simulink model "DIPCRT"  (R2015a)
settings: Solver=ode23  SolverMode=SingleTasking  StartTime=0.0  StopTime=3  FixedStep=1e-3  RelTol=1e-3
values from neighbouring files (symbols this model uses):
  deltas = 1000    [DIPCRTinit.m]
  deltav = 5000    [DIPCRTinit.m]
  ds = 1000    [DIPCRTinit.m]
  dv = 5000    [DIPCRTinit.m]
  g = [0;0;0]    [DIPCRTinit.m]
  j0 = 1    [DIPCRTinit.m]
  j1 = 10    [DIPCRTinit.m]
  j2 = 10    [DIPCRTinit.m]
  j3 = 10    [DIPCRTinit.m]
  j4 = 10    [DIPCRTinit.m]
  jv = 1    [DIPCRTinit.m]
  kappas = 2000    [DIPCRTinit.m]
  kappav = 20000    [DIPCRTinit.m]
  kpr = 500    [DIPCRTinit.m]
  kpt = 500    [DIPCRTinit.m]
  ks = 2000    [DIPCRTinit.m]
  kv = 30    [DIPCRTinit.m]
  m0 = 10    [DIPCRTinit.m]
  m1 = 10    [DIPCRTinit.m]
  m2 = 10    [DIPCRTinit.m]
  m3 = 10    [DIPCRTinit.m]
  m4 = 10    [DIPCRTinit.m]
  mv = 10    [DIPCRTinit.m]
libraries: aerolibutil x22, dspinverses x3, aerolibtransform2 x2, simulink x2
(part 2 of 2)

== matlab function DIPCRT/Interaction dynamics1/MATLAB Function ==
  data: r parameter; A output; x input
function A = ConstraintMatrix(r,x)
A = [-eye(3) skew_sm(quatrot(x(4:7),r(1:3))) eye(3) zeros(3,21);
        zeros(3) -eye(3) zeros(3) eye(3) zeros(3,18);
        -eye(3) skew_sm(quatrot(x(4:7),r(4:6))) zeros(3,6) eye(3) zeros(3,15);
        zeros(3) -eye(3) zeros(3,9) eye(3) zeros(3,12);
        -eye(3) skew_sm(quatrot(x(4:7),r(7:9))) zeros(3,12) eye(3) zeros(3,9);
        zeros(3) -eye(3) zeros(3,15) eye(3) zeros(3,6);
        -eye(3) skew_sm(quatrot(x(4:7),r(10:12))) zeros(3,18) eye(3) zeros(3);
        zeros(3) -eye(3) zeros(3,21) eye(3)];

== matlab function DIPCRT/Interaction dynamics1/Centripetal Force ==
  data: dx input; b output; r parameter; x input
function b = centripetalforce(dx,r,x)
b = [skew_sm(dx(4:6))*skew_sm(dx(4:6))*quatrot(x(4:7),r(1:3));
     zeros(3,1);
     skew_sm(dx(4:6))*skew_sm(dx(4:6))*quatrot(x(4:7),r(4:6));
     zeros(3,1);
     skew_sm(dx(4:6))*skew_sm(dx(4:6))*quatrot(x(4:7),r(7:9));
     zeros(3,1);
     skew_sm(dx(4:6))*skew_sm(dx(4:6))*quatrot(x(4:7),r(10:12));
     zeros(3,1)];

== matlab function DIPCRT/Interaction dynamics1/Coriolis Force ==
  data: dx input; hcoriolis output; j0 parameter; m0 parameter
function hcoriolis = CoriolisForce(dx,j0,m0)
hcoriolis = [m0*skew_sm(dx(4:6))*dx(1:3);
        j0*skew_sm(dx(4:6))*dx(4:6)];

== matlab function DIPCRT/Manipulator Springs/Spring 1/MATLAB Function1 ==
  data: eta input; K output; ks parameter; kappas parameter
function K = stiffness(eta,ks,kappas)
K = blkdiag(ks*eye(3),2*eta*kappas*eye(3));

== matlab function DIPCRT/Manipulator Springs/Spring 2/MATLAB Function1 ==
  data: eta input; K output; ks parameter; kappas parameter
function K = stiffness(eta,ks,kappas)
K = blkdiag(ks*eye(3),2*eta*kappas*eye(3));

== matlab function DIPCRT/Manipulator Springs/Spring 3/MATLAB Function1 ==
  data: eta input; K output; ks parameter; kappas parameter
function K = stiffness(eta,ks,kappas)
K = blkdiag(ks*eye(3),2*eta*kappas*eye(3));

== matlab function DIPCRT/Manipulator Springs/Spring 4/MATLAB Function1 ==
  data: eta input; K output; ks parameter; kappas parameter
function K = stiffness(eta,ks,kappas)
K = blkdiag(ks*eye(3),2*eta*kappas*eye(3));

== matlab function DIPCRT/Virtual Object Simulation/Grasp Matrix ==
  data: rv parameter; G output; x input
function G = GraspMatrix(rv,x)
G = [eye(3) zeros(3) eye(3) zeros(3) eye(3) zeros(3) eye(3) zeros(3);
    skew_sm(quatrot(x(4:7),rv(1:3))) eye(3) skew_sm(quatrot(x(4:7),rv(4:6))) eye(3) skew_sm(quatrot(x(4:7),rv(7:9))) eye(3) skew_sm(quatrot(x(4:7),rv(10:12))) eye(3)];

== matlab function DIPCRT/Virtual Object Simulation/Coriolis Force ==
  data: dx input; hcoriolis output; j0 parameter; m0 parameter
function hcoriolis = CoriolisForce(dx,j0,m0)
hcoriolis = [m0*skew_sm(dx(4:6))*dx(1:3);
        j0*skew_sm(dx(4:6))*dx(4:6)];

== matlab function DIPCRT/Virtual Object Erhart/Centripetal Force ==
  data: dx input size=6; b output; rv parameter; x input size=7
function b = centripetalforce(dx,rv,x)
b = [skew_sm(dx(4:6))*skew_sm(dx(4:6))*quatrot(x(4:7),rv(1:3));
     zeros(3,1);
     skew_sm(dx(4:6))*skew_sm(dx(4:6))*quatrot(x(4:7),rv(4:6));
     zeros(3,1);
     skew_sm(dx(4:6))*skew_sm(dx(4:6))*quatrot(x(4:7),rv(7:9));
     zeros(3,1);
     skew_sm(dx(4:6))*skew_sm(dx(4:6))*quatrot(x(4:7),rv(10:12));
     zeros(3,1)];

== matlab function DIPCRT/Virtual Object Erhart/Coriolis Force ==
  data: dx input; hcoriolis output; j0 parameter; m0 parameter
function hcoriolis = CoriolisForce(dx,j0,m0)
hcoriolis = [m0*skew_sm(dx(4:6))*dx(1:3);
        j0*skew_sm(dx(4:6))*dx(4:6)];

== matlab function DIPCRT/Virtual Object Erhart/MATLAB Function ==
  data: rv parameter; A output; x input
function A = ConstraintMatrix(rv,x)
A = [-eye(3) skew_sm(quatrot(x(4:7),rv(1:3))) eye(3) zeros(3,21);
        zeros(3) -eye(3) zeros(3) eye(3) zeros(3,18);
        -eye(3) skew_sm(quatrot(x(4:7),rv(4:6))) zeros(3,6) eye(3) zeros(3,15);
        zeros(3) -eye(3) zeros(3,9) eye(3) zeros(3,12);
        -eye(3) skew_sm(quatrot(x(4:7),rv(7:9))) zeros(3,12) eye(3) zeros(3,9);
        zeros(3) -eye(3) zeros(3,15) eye(3) zeros(3,6);
        -eye(3) skew_sm(quatrot(x(4:7),rv(10:12))) zeros(3,18) eye(3) zeros(3);
        zeros(3) -eye(3) zeros(3,21) eye(3)];

== matlab function DIPCRT/Manipulator Springs/Grasp Matrix ==
  data: rv parameter; G output; x input
function G = GraspMatrix(rv,x)
G = [eye(3) zeros(3) eye(3) zeros(3) eye(3) zeros(3) eye(3) zeros(3);
    skew_sm(quatrot(x(4:7),rv(1:3))) eye(3) skew_sm(quatrot(x(4:7),rv(4:6))) eye(3) skew_sm(quatrot(x(4:7),rv(7:9))) eye(3) skew_sm(quatrot(x(4:7),rv(10:12))) eye(3)];

== matlab function DIPCRT/Manipulator Springs/Spring 2/Coriolis Force1 ==
  data: dx input; hcoriolis output; j1 parameter; m1 parameter
function hcoriolis = CoriolisForce(dx,j1,m1)
hcoriolis = [m1*skew_sm(dx(4:6))*dx(1:3);
        j1*skew_sm(dx(4:6))*dx(4:6)];

== matlab function DIPCRT/Manipulator Springs/Spring 3/Coriolis Force1 ==
  data: dx input; hcoriolis output; j1 parameter; m1 parameter
function hcoriolis = CoriolisForce(dx,j1,m1)
hcoriolis = [m1*skew_sm(dx(4:6))*dx(1:3);
        j1*skew_sm(dx(4:6))*dx(4:6)];

== matlab function DIPCRT/Manipulator Springs/Spring 1/Coriolis Force1 ==
  data: dx input; hcoriolis output; j1 parameter; m1 parameter
function hcoriolis = CoriolisForce(dx,j1,m1)
hcoriolis = [m1*skew_sm(dx(4:6))*dx(1:3);
        j1*skew_sm(dx(4:6))*dx(4:6)];

== matlab function DIPCRT/Manipulator Springs/Spring 4/Coriolis Force1 ==
  data: dx input; hcoriolis output; j1 parameter; m1 parameter
function hcoriolis = CoriolisForce(dx,j1,m1)
hcoriolis = [m1*skew_sm(dx(4:6))*dx(1:3);
        j1*skew_sm(dx(4:6))*dx(4:6)];

== matlab function DIPCRT/Local Force Control/Subsystem/Subsystem/k1; 2kappa1*eta1 ==
  data: eta1 input; kpt parameter; kpr parameter; K output
function K = stiffness(eta1,kpt,kpr)
K = blkdiag(kpt*eye(3),2*eta1*kpr*eye(3));

== matlab function DIPCRT/Local Force Control/Subsystem/Subsystem1/k1; 2kappa1*eta2 ==
  data: eta2 input; kpt parameter; K output; kpr parameter
function K = stiffness(eta2,kpt,kpr)
K = blkdiag(kpt*eye(3),2*eta2*kpr*eye(3));

== matlab function DIPCRT/Object Spring/MATLAB Function1 ==
  data: eta input; K output; kv parameter; kappav parameter
function K = stiffness(eta,kv,kappav)
% if energy>100
%     energy=100;
% % elseif energy<0
% %     energy=0;
% end
%K = blkdiag(kv*energy/100*eye(3),2*eta*kappav*energy/100*eye(3));
K = blkdiag(kv*eye(3),2*eta*kappav*eye(3));

== matlab function DIPCRT/Local Force Control/Subsystem/Subsystem2/k1; 2kappa1*eta3 ==
  data: eta3 input; kpt parameter; K output; kpr parameter
function K = stiffness(eta3,kpt,kpr)
K = blkdiag(kpt*eye(3),2*eta3*kpr*eye(3));

== matlab function DIPCRT/Local Force Control/Subsystem/Subsystem3/k1; 2kappa1*eta4 ==
  data: eta4 input; kpt parameter; K output; kpr parameter
function K = stiffness(eta4,kpt,kpr)
K = blkdiag(kpt*eye(3),2*eta4*kpr*eye(3));

== matlab function DIPCRT/Manipulator dynamics/Reduced Constraint Matrix ==
  data: r parameter; Ared output; x input
function Ared = ReducedConstraintMAtrix(r,x)
Ared = [-eye(3) skew_sm(quatrot(x(4:7),r(4:6)-r(1:3))) eye(3) zeros(3,15);
        zeros(3) -eye(3) zeros(3) eye(3) zeros(3,12);
        -eye(3) skew_sm(quatrot(x(4:7),r(7:9)-r(1:3))) zeros(3,6) eye(3) zeros(3,9);
        zeros(3) -eye(3) zeros(3,9) eye(3) zeros(3,6);
        -eye(3) skew_sm(quatrot(x(4:7),r(10:12)-r(1:3))) zeros(3,12) eye(3) zeros(3);
        zeros(3) -eye(3) zeros(3,15) eye(3)];

== matlab function DIPCRT/Manipulator dynamics/Centripal Force ==
  data: r parameter; x input; bred output; dx input
function bred = ReducedCentripetalvector(r,x,dx)
bred = [skew_sm(dx(4:6))*skew_sm(dx(4:6))*quatrot(x(4:7),(r(4:6)-r(1:3)));
        zeros(3,1);
        skew_sm(dx(4:6))*skew_sm(dx(4:6))*quatrot(x(4:7),(r(7:9)-r(1:3)));
        zeros(3,1);
        skew_sm(dx(4:6))*skew_sm(dx(4:6))*quatrot(x(4:7),(r(10:12)-r(1:3)));
        zeros(3,1)];

== matlab function DIPCRT/Manipulator motion/Grasp Matrix ==
  data: r parameter; G output; x input
function G = GraspMatrix(r,x)
G = [eye(3) zeros(3) eye(3) zeros(3) eye(3) zeros(3) eye(3) zeros(3);
    skew_sm(quatrot(x(4:7),r(1:3))) eye(3) skew_sm(quatrot(x(4:7),r(4:6))) eye(3) skew_sm(quatrot(x(4:7),r(7:9))) eye(3) skew_sm(quatrot(x(4:7),r(10:12))) eye(3)];

== matlab function DIPCRT/Manipulator motion/Manipualtor pose in world frame ==
  data: p_o input; q_o input size=4; x output; r parameter
function x = manipulatorpose(p_o,q_o,r)

x = [p_o + quatrot(q_o,r(1:3));
        q_o;
        p_o + quatrot(q_o,r(4:6));
        q_o;
        p_o + quatrot(q_o,r(7:9));
        q_o;
        p_o + quatrot(q_o,r(10:12));
        q_o ];

== matlab function DIPCRT/Manipulator dynamics/World to Object Frame ==
  data: hw input; x input; h_int output
function h_int = inertial2objectFrame(hw,x)

h_int = [quatrot(quatconj(x(4:7)')',hw(1:3));
         hw(4:6);%quatrot(quatconj(x(4:7)')',hw(4:6));
         quatrot(quatconj(x(4:7)')',hw(7:9));
         hw(10:12);%quatrot(quatconj(x(4:7)')',hw(10:12));
         quatrot(quatconj(x(4:7)')',hw(13:15));
         hw(16:18);%quatrot(quatconj(x(4:7)')',hw(16:18));
         quatrot(quatconj(x(4:7)')',hw(19:21));
         hw(22:24)];%quatrot(quatconj(x(4:7)')',hw(22:24));];
